simulink model "BacStaphPhage2021aModel-2"  (R2024a)
settings: Solver=ode1  StartTime=0.0  StopTime=15  FixedStep=0.001  RelTol=1e-3
settings Model: Creator=caran  LastModifiedBy=claudelieber
settings SolverCC: AlgebraicLoopSolver=TrustRegion
settings OptimizationCC: ReuseModelBlockBuffer=off
settings DebuggingCC: UnconnectedInputMsg=warning  UnconnectedOutputMsg=warning  UnconnectedLineMsg=warning
settings ModelReferenceCC: EnableRefExpFcnMdlSchedulingChecks=on
settings RTWCC: GPUComputeCapability=3.5  DLArmComputeVersion=19.05

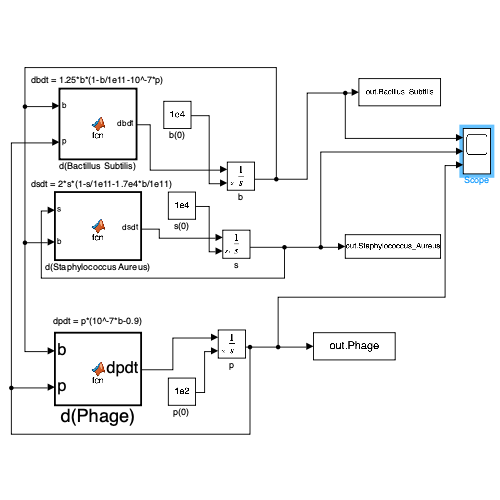
[thumbnail: Simulink's stored preview of the top-level diagram]
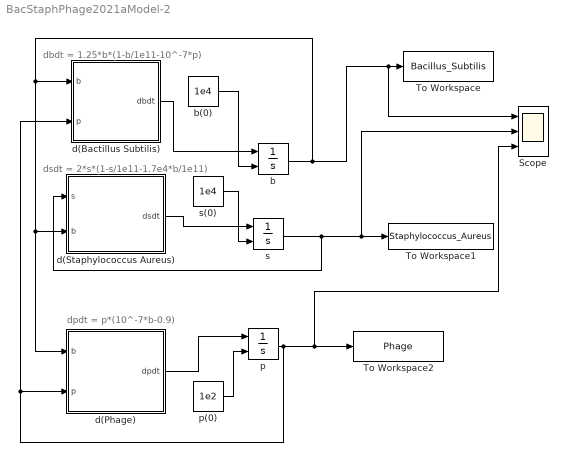
== system BacStaphPhage2021aModel-2 ==
  note: dpdt = p*(10^-7*b-0.9)
  note: dsdt = 2*s*(1-s/1e11-1.7e4*b/1e11)
  note: dbdt = 1.25*b*(1-b/1e11-10^-7*p)
  Scope : Scope  NumInputPorts=3
  To Workspace : ToWorkspace  VariableName=Bacillus_Subtilis  SampleTime=-1
  To Workspace1 : ToWorkspace  VariableName=Staphylococcus_Aureus  SampleTime=-1
  To Workspace2 : ToWorkspace  VariableName=Phage  SampleTime=-1
  b : Integrator  InitialConditionSource=external
  b(0) : Constant  Value=1e4
  d(Bactillus Subtilis) : MATLAB Function  TreatAsAtomicUnit=on
  d(Phage) : MATLAB Function  TreatAsAtomicUnit=on
  d(Staphylococcus Aureus) : MATLAB Function  TreatAsAtomicUnit=on
  p : Integrator  InitialConditionSource=external
  p(0) : Constant  Value=1e2
  s : Integrator  InitialConditionSource=external
  s(0) : Constant  Value=1e4
  wires:
  b/1 -> d(Bactillus Subtilis)/1(b), d(Staphylococcus Aureus)/2(b), d(Phage)/1(b), Scope/1, To Workspace/1
  s/1 -> d(Staphylococcus Aureus)/1(s), Scope/2, To Workspace1/1
  p/1 -> d(Phage)/2(p), d(Bactillus Subtilis)/2(p), To Workspace2/1, Scope/3
  s(0)/1 -> s/2
  d(Staphylococcus Aureus)/1(dsdt) -> s/1
  b(0)/1 -> b/2
  d(Bactillus Subtilis)/1(dbdt) -> b/1
  d(Phage)/1(dpdt) -> p/1
  p(0)/1 -> p/2

== matlab function BacStaphPhage2021aModel-2/d(Staphylococcus Aureus) ==
  data: s input; b input; dsdt output
function dsdt = fcn(s,b)

dsdt = 2*s*(1-s/1e11-1.7e4*b/1e11);

== matlab function BacStaphPhage2021aModel-2/d(Bactillus Subtilis) ==
  data: b input; p input; dbdt output
function dbdt = fcn(b,p)

dbdt = 1.25*b*(1-b/1e11-10^-7*p);

== matlab function BacStaphPhage2021aModel-2/d(Phage) ==
  data: b input; dpdt output; p input
function dpdt = fcn(b,p)

dpdt = p*(1e-7*b-0.9);
